simulink model "modeloProcessoAula5"  (R2020b)
settings: Solver=VariableStepAuto  StartTime=0.0  StopTime=400  RelTol=1e-3
values from neighbouring files (symbols this model uses):
  u0 = 52433    [script.m]
  y0 = 40982    [script.m]
libraries: cstblocks x4, pid_lib x1
settings Model: Creator=Victor  LastModifiedBy=Victor

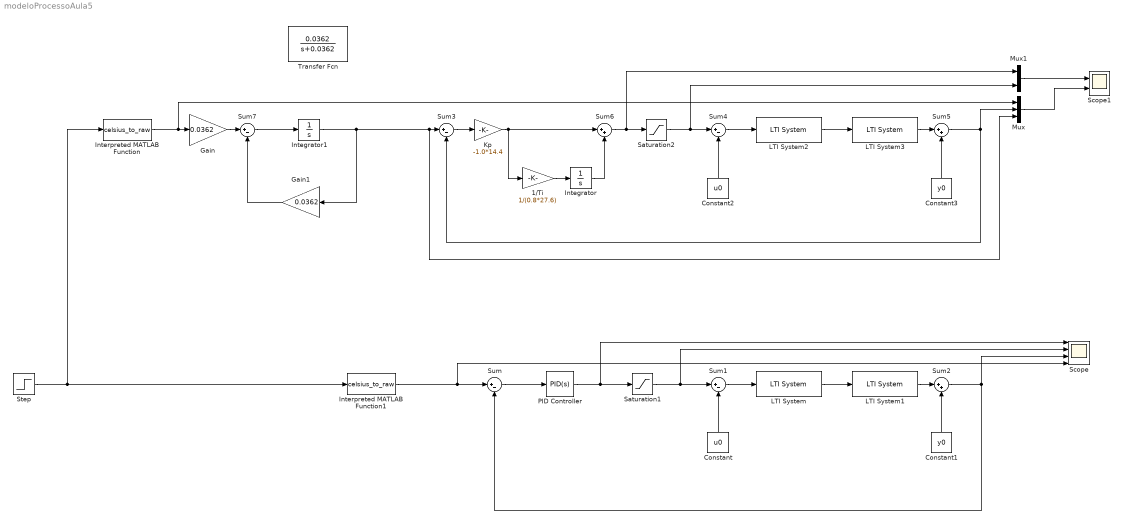
== system modeloProcessoAula5 ==
  1/Ti : Gain  Gain=1/(0.8*27.6)
  Constant : Constant  Value=u0
  Constant1 : Constant  Value=y0
  Constant2 : Constant  Value=u0
  Constant3 : Constant  Value=y0
  Gain : Gain  Gain=0.0362
  Gain1 : Gain  Gain=0.0362
  Integrator : Integrator  InitialCondition=54000
  Integrator1 : Integrator  InitialCondition=41000
  Interpreted MATLAB Function : MATLABFcn  MATLABFcn=celsius_to_raw
  Interpreted MATLAB Function1 : MATLABFcn  MATLABFcn=celsius_to_raw
  Kp : Gain  Gain=-1.0*14.4
  LTI System : cstblocks/LTI System  sys=G  IC=[]
  LTI System1 : cstblocks/LTI System  sys=F  IC=[]
  LTI System2 : cstblocks/LTI System  sys=G  IC=[]
  LTI System3 : cstblocks/LTI System  sys=F  IC=[]
  Mux : Mux  Inputs=3
  Mux1 : Mux  Inputs=2
  PID Controller : pid_lib/PID Controller  Controller=PID  Form=Parallel  TimeDomain=Continuous-time  UseExternalTs=off  SampleTime=-1  IntegratorMethod=Forward Euler  FilterMethod=Forward Euler  ControllerParametersSource=internal  P=-10.2665274576316  I=-0.304233974069868  D=-48.1029394945244  UseFilter=on  N=0.116585307006618  TunerSelectOption=Transfer Function Based (PID Tuner App)  InitialConditionSource=internal  InitialConditionForIntegrator=0  InitialConditionForFilter=0  DifferentiatorICPrevScaledInput=0  ExternalReset=none  TrackingMode=off  Kt=1  LimitOutput=off  SatLimitsSource=internal  UpperSaturationLimit=inf  LowerSaturationLimit=-inf  LinearizeAsGain=on  AntiWindupMode=none  Kb=1  POutMin=[]  POutMax=[]  IOutMin=[]  IOutMax=[]  DOutMin=[]  DOutMax=[]  NOutMin=[]  NOutMax=[]  SumOutMin=[]  SumOutMax=[]  SaturationOutMin=[]  SaturationOutMax=[]  PParamMin=[]  PParamMax=[]  IParamMin=[]  IParamMax=[]  DParamMin=[]  DParamMax=[]  NParamMin=[]  NParamMax=[]  KbParamMin=[]  KbParamMax=[]  KtParamMin=[]  KtParamMax=[]  KbOutMin=[]  KbOutMax=[]  KtOutMin=[]  KtOutMax=[]  IntegratorOutMin=[]  IntegratorOutMax=[]  FilterOutMin=[]  FilterOutMax=[]  SumI1OutMin=[]  SumI1OutMax=[]  SumI2OutMin=[]  SumI2OutMax=[]  SumI3OutMin=[]  SumI3OutMax=[]  SumI4OutMin=[]  SumI4OutMax=[]  SumDOutMin=[]  SumDOutMax=[]  DifferentiatorOutMin=[]  DifferentiatorOutMax=[]  FilterDiffOutCoefMin=[]  FilterDiffOutCoefMax=[]  ReciprocalOutMin=[]  ReciprocalOutMax=[]  SumDenOutMin=[]  SumDenOutMax=[]  SumNumOutMin=[]  SumNumOutMax=[]  DivideOutMin=[]  DivideOutMax=[]  UdiffTsProdOutMin=[]  UdiffTsProdOutMax=[]  NTsProdOutMin=[]  NTsProdOutMax=[]  UintegralTsProdOutMin=[]  UintegralTsProdOutMax=[]  UngainTsProdOutMin=[]  UngainTsProdOutMax=[]  IntegratorContinuousStateAttributes=''  IntegratorStateMustResolveToSignalObject=off  IntegratorRTWStateStorageClass=Auto  FilterContinuousStateAttributes=''  FilterStateMustResolveToSignalObject=off  FilterRTWStateStorageClass=Auto  ParallelPVariant=InternalParameters  IdealPVariant=Disabled  IVariant=InternalParameters  DVariant=InternalParameters  IntegratorVariant=Continuous  SatVariant=Disabled  AWVariant=Passthrough  PCopyVariant=Disabled  TRVariant=Disabled  FdbkBlocksVariant=Forward  IdealPFdbkVariant=Disabled  SatFdbkVariant=Disabled  DerivativeFilterVariant=ContFilter  NVariant=InternalParameters  NCopyVariant=Disabled  FilterICVariant=InternalICsFilter  IntegratorICVariant=InternalICs  ExternalResetVariant=Disabled  TRSumVariant=Passthrough  SumFdbkVariant=Disabled  SumVariant=Sum_PID  TsampFilterVariant=InternalTs  TsampNgainVariant=Passthrough  TsampIntegralVariant=Passthrough  ExternalSaturationOutDataTypeStr=Inherit: Same as second input
  Saturation1 : Saturate  UpperLimit=65535  LowerLimit=32786
  Saturation2 : Saturate  UpperLimit=65535  LowerLimit=32786
  Scope : Scope  NumInputPorts=4
  Scope1 : Scope  NumInputPorts=2
  Step : Step  Time=100  Before=29.5  After=34.5  SampleTime=0
  Sum{,1,3..4,7} (5 alike) : Sum  Inputs=|+-
  Sum2 : Sum  Inputs=|++
  Sum5 : Sum  Inputs=|++
  Sum6 : Sum  Inputs=|++
  Transfer Fcn : TransferFcn  Numerator=[ 0.0362]  Denominator="[1  0.0362]"
  wires:
  Constant/1 -> Sum1/2
  Constant1/1 -> Sum2/2
  Saturation1/1 -> Scope/2, Sum1/1
  Sum1/1 -> LTI System/1
  Sum2/1 -> Sum/2, Scope/3
  LTI System1/1 -> Sum2/1
  LTI System/1 -> LTI System1/1
  Interpreted MATLAB Function1/1 -> Scope/4, Sum/1
  Sum/1 -> PID Controller/1
  PID Controller/1 -> Scope/1, Saturation1/1
  Interpreted MATLAB Function/1 -> Mux/1, Gain/1
  LTI System3/1 -> Sum5/1
  Constant2/1 -> Sum4/2
  LTI System2/1 -> LTI System3/1
  Constant3/1 -> Sum5/2
  Saturation2/1 -> Mux1/2, Sum4/1
  Sum4/1 -> LTI System2/1
  Sum6/1 -> Mux1/1, Saturation2/1
  Sum3/1 -> Kp/1
  Step/1 -> Interpreted MATLAB Function1/1, Interpreted MATLAB Function/1
  Kp/1 -> 1/Ti/1, Sum6/1
  1/Ti/1 -> Integrator/1
  Integrator/1 -> Sum6/2
  Sum5/1 -> Mux/2, Sum3/2
  Mux/1 -> Scope1/2
  Mux1/1 -> Scope1/1
  Integrator1/1 -> Mux/3, Sum3/1, Gain1/1
  Gain/1 -> Sum7/1
  Sum7/1 -> Integrator1/1
  Gain1/1 -> Sum7/2
